simulink model "tengbeudpv1"  (Simulink 7.4)
settings: Solver=ode45  StartTime=0.0  StopTime=1000  RelTol=1e-3
libraries: xbsIndex_r4 x132, xps_library x15, casper_library_misc x6, casper_library_flow_control x4
settings Model: Creator=dsp  LastModifiedBy=gofrito  CovModelRefEnable=off
settings OptimizationCC: InitFltsAndDblsToZero=on
settings DebuggingCC: SaveWithParameterizedLinksMsg=none  SignalResolutionControl=TryResolveAllWithWarning  MultiTaskDSMMsg=warning  MultiTaskCondExecSysMsg=none  StrictBusMsg=None
settings RTWCC: IncludeERTFirstTime=on
settings GRTTargetCC: TargetFcnLib=ansi_tfl_tmw.mat

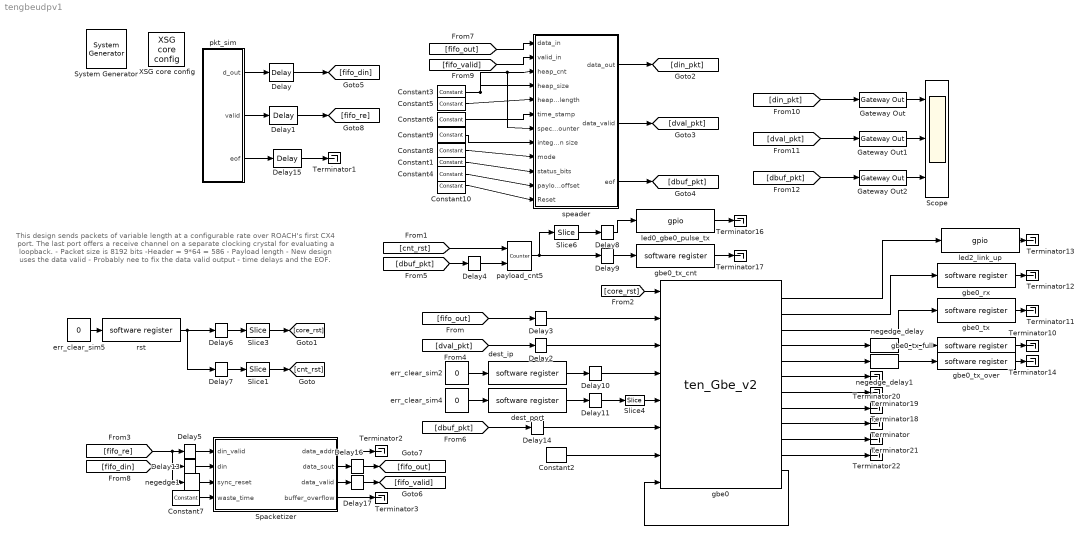
== system tengbeudpv1 ==
  note: This design sends packets of variable length at a configurable rate
      | over ROACH's first CX4 port.
      | The last port offers a receive channel on a separate
      | clocking crystal for evaluating a loopback.
      |
      | - Packet size is 8192 bits
      | -Header = 9*64 = 586
      | - Payload length
      | - New design uses the data valid
      | - Probably nee to fix the data valid output - time delays and the EOF.
  " System Generator" : xbsIndex_r4/ System Generator  Tag=genX  SystemSampleTime=-1  xilinxfamily=virtex5  part=xc5vsx95t  speed=-1  package=ff1136  synthesis_tool=XST  clock_wrapper=Clock Enables  directory=./tengbeudpv1/sysgen  testbench=off  simulink_period=1  sysclk_period=5  dcm_input_clock_period=100  incr_netlist=off  trim_vbits=Everywhere in SubSystem  dbl_ovrd=According to Block Masks  core_generation=According to Block Masks  run_coregen=off  deprecated_control=off  eval_field=0  block_type=sysgen
      settings: block_version=10.1.3
  Constant{1,4,6,8..9} (5 alike) : xbsIndex_r4/Constant  arith_type=Unsigned  const=0  n_bits=40  bin_pt=0  explicit_period=on  period=1  equ=P=C  opselect=C  inp2=PCIN>>17  opr=+  inp1=P  carry=CIN  dbl_ovrd=off  block_type=constant
  Constant10 : xbsIndex_r4/Constant  arith_type=Boolean  const=0  n_bits=40  bin_pt=0  explicit_period=on  period=1  equ=P=C  opselect=C  inp2=PCIN>>17  opr=+  inp1=P  carry=CIN  dbl_ovrd=off  block_type=constant
  Constant2 : xbsIndex_r4/Constant  arith_type=Boolean  const=1  n_bits=1  bin_pt=0  explicit_period=on  period=1  equ=P=C  opselect=C  inp2=PCIN>>17  opr=+  inp1=P  carry=CIN  dbl_ovrd=off  block_type=constant
  Constant3 : xbsIndex_r4/Constant  arith_type=Unsigned  const=128*2+6*8  n_bits=40  bin_pt=0  explicit_period=on  period=1  equ=P=C  opselect=C  inp2=PCIN>>17  opr=+  inp1=P  carry=CIN  dbl_ovrd=off  block_type=constant
  Constant5 : xbsIndex_r4/Constant  arith_type=Unsigned  const=256  n_bits=40  bin_pt=0  explicit_period=on  period=1  equ=P=C  opselect=C  inp2=PCIN>>17  opr=+  inp1=P  carry=CIN  dbl_ovrd=off  block_type=constant
  Constant7 : xbsIndex_r4/Constant  arith_type=Unsigned  const=4  n_bits=7  bin_pt=0  explicit_period=on  period=1  equ=P=C  opselect=C  inp2=PCIN>>17  opr=+  inp1=P  carry=CIN  dbl_ovrd=off  block_type=constant
  Delay{,1,4,6..11,15..17} (12 alike) : xbsIndex_r4/Delay  en=off  latency=4  dbl_ovrd=off  reg_retiming=off  block_type=delay
      settings: block_version=11.4
  Delay{2,5,13..14} (4 alike) : xbsIndex_r4/Delay  en=off  latency=2  dbl_ovrd=off  reg_retiming=off  block_type=delay
      settings: block_version=11.4
  Delay3 : xbsIndex_r4/Delay  en=off  latency=3  dbl_ovrd=off  reg_retiming=off  block_type=delay
      settings: block_version=11.4
  Gateway Out : xbsIndex_r4/Gateway Out  hdl_port=on  timing_constraint=None  locs_specified=off  LOCs={}  block_type=gatewayout
      settings: infoedit="Gateway out block.  Converts Xilinx fixed point inputs into ouputs of type Simulink integer, double, or fixed point.<br><br>Hardware notes:  In hardware these blocks become top level output ports or are discarded, depending on how they are configured."  block_version=11.4
  Gateway Out1 : xbsIndex_r4/Gateway Out  hdl_port=on  timing_constraint=None  locs_specified=off  LOCs={}  block_type=gatewayout
      settings: infoedit="Gateway out block.  Converts Xilinx fixed point inputs into ouputs of type Simulink integer, double, or fixed point.<br><br>Hardware notes:  In hardware these blocks become top level output ports or are discarded, depending on how they are configured."  block_version=11.4
  Gateway Out2 : xbsIndex_r4/Gateway Out  hdl_port=on  timing_constraint=None  locs_specified=off  LOCs={}  block_type=gatewayout
      settings: infoedit="Gateway out block.  Converts Xilinx fixed point inputs into ouputs of type Simulink integer, double, or fixed point.<br><br>Hardware notes:  In hardware these blocks become top level output ports or are discarded, depending on how they are configured."  block_version=11.4
  Scope : Scope  NumInputPorts=3
      settings: YMin=-5~-5~-5  YMax=5~5~5
  Slice1 : xbsIndex_r4/Slice  nbits=1  boolean_output=on  mode=Lower Bit Location + Width  bit1=0  base1=MSB of Input  bit0=0  base0=LSB of Input  dbl_ovrd=off  block_type=slice
      settings: infoedit="Extracts a given range of bits from each input sample and presents it at the output.  The output type is ordinarily unsigned with binary point at zero, but can be Boolean when the slice is one bit wide.<P><P>Hardware notes: In hardware this block costs nothing."  block_version=10.1.3
  Slice3 : xbsIndex_r4/Slice  nbits=1  boolean_output=on  mode=Lower Bit Location + Width  bit1=0  base1=MSB of Input  bit0=1  base0=LSB of Input  dbl_ovrd=off  block_type=slice
      settings: block_version=10.1.3
  Slice4 : xbsIndex_r4/Slice  nbits=16  boolean_output=off  mode=Lower Bit Location + Width  bit1=0  base1=MSB of Input  bit0=0  base0=LSB of Input  dbl_ovrd=off  block_type=slice
      settings: infoedit="Extracts a given range of bits from each input sample and presents it at the output.  The output type is ordinarily unsigned with binary point at zero, but can be Boolean when the slice is one bit wide.<P><P>Hardware notes: In hardware this block costs nothing."  block_version=10.1.3
  Slice6 : xbsIndex_r4/Slice  nbits=1  boolean_output=on  mode=Lower Bit Location + Width  bit1=0  base1=MSB of Input  bit0=27-12  base0=LSB of Input  dbl_ovrd=off  block_type=slice
      settings: infoedit="Extracts a given range of bits from each input sample and presents it at the output.  The output type is ordinarily unsigned with binary point at zero, but can be Boolean when the slice is one bit wide.<P><P>Hardware notes: In hardware this block costs nothing."  block_version=10.1.3
  Spacketizer : Subsystem  AncestorBlock=gbt_library/Spacketizer  mask(packetizer){pin_width=256, sout_width=64, fifo_depth=2K, total_words=32}
      mask prompts: pin_width "Parallel Input Width"; sout_width "Serial Output Width"; fifo_depth "FIFO depth"; total_words "Total number of data points"
      mask help:
      | This block is intended to serialize data that is 'bursty', that is,
      | the average data rate is small but per cycle the data is highly
      | parallel and can contain many points simultaneously.  This situation
      | is common with the streaming CASPER FFTs and related blocks.
      |
      | The serialization buffers the data when valid and independently
      | serializes the data when the buffer is non-empty.  For convenience, the
      | data is counted as it is serialized and signals exist to indicate
      | that the serial output is valid or that a buffer overflow has occured.  The
      | block will not stop in the case of an overflow, and the overflow
      | signal is not held high after it occurs.
      |
      | For example usage, see 'roach_spec_2adc_borph' in 'SVNROOT/trunk/projects/roach_spec/'
      | or the test case in 'SVNROOT/trunk/mlib_devel_10_1/Tests/packetizer_test.mdl'
      |
      | For extended documentation, please see the CASPER wiki
      mask init:
      | packetizer_init(gcb, 'pin_width', pin_width, 'sout_width', sout_width, 'total_words', total_words, 'fifo_depth', fifo_depth)
      | % packetizer_init(gcb, ...
      | %     'pin_width', pin_width, ...
      | %     'sout_width', sout_width, ...
      | %   %  'fifo_depth', fifo_depth, ...
      | %     'total_words', total_words);
      settings: AttributesFormatString=|
      | Parallel Input Width: 256
      | Serial Output Width: 64
      mask StyleString: edit,edit,popup(16|32|64|128|256|512|1K|2K|4K|8K|16K|32K|64K),edit
  Terminator{,1..3,10..14,16..22} (16 alike) : Terminator
  XSG core config : xps_library/XSG core config  Tag=xps:xsg  SystemSampleTime=-1  hw_sys=ROACH:sx95t  ibob_linux=off  clk_src=sys_clk2x  iBOB_clk_src=sys_clk  BEE2_ctrl_clk_src=sys_clk  BEE2_usr_clk_src=sys_clk  ROACH_clk_src=sys_clk2x  CORR_clk_src=sys_clk  gpio_clk_io_group=iBOB:sma  gpio_clk_bit_index=0  clk_rate=200  sample_period=1  synthesis_tool=XST  mpc_type=powerpc440_ext
  dest_ip : xps_library/software register  Tag=xps:sw_reg  SystemSampleTime=-1  io_dir=From Processor  arith_type=Unsigned  bitwidth=32  bin_pt=0  sample_period=1  gw_name=tengbeudpv1_dest_ip_user_data_out
      link override r_10gbe_demo_dest_ip_user_data_out: arith_type=Unsigned  n_bits=32  bin_pt=0  period=1
      link override r_10gbe_test_dest_ip_user_data_out: arith_type=Unsigned  n_bits=32  bin_pt=0  period=1
      link override r_xaui_test_cnt_rst_user_data_out: arith_type=Unsigned  n_bits=32  bin_pt=0  period=1
  dest_port : xps_library/software register  Tag=xps:sw_reg  SystemSampleTime=-1  io_dir=From Processor  arith_type=Unsigned  bitwidth=32  bin_pt=0  sample_period=1  gw_name=tengbeudpv1_dest_port_user_data_out
      link override r_10gbe_demo_dest_port_user_data_out: arith_type=Unsigned  n_bits=32  bin_pt=0  period=1
      link override r_10gbe_test_dest_port_user_data_out: arith_type=Unsigned  n_bits=32  bin_pt=0  period=1
      link override r_xaui_test_cnt_rst_user_data_out: arith_type=Unsigned  n_bits=32  bin_pt=0  period=1
  err_clear_sim2 : Constant  Value=0  OutDataType=sfix(16)  OutScaling=2^0
  err_clear_sim4 : Constant  Value=0  OutDataType=sfix(16)  OutScaling=2^0
  err_clear_sim5 : Constant  Value=0  OutDataType=sfix(16)  OutScaling=2^0
  gbe0 : xps_library/ten_Gbe_v2  Tag=xps:tengbe_v2  SystemSampleTime=-1  port=0  rx_dist_ram=off  large_frames=on  show_param=on  pre_emph=3  swing=800  fab_en=on  fab_mac=hex2dec('123456780000')  fab_ip=10*(2^24) + 0*(2^16) + 0*(2^8) + 20*(2^0)  fab_udp=10000  fab_gate=1  cpu_rx_en=on  cpu_tx_en=on
  gbe0_rx : xps_library/software register  Tag=xps:sw_reg  SystemSampleTime=-1  io_dir=To Processor  arith_type=Unsigned  bitwidth=32  bin_pt=0  sample_period=1  gw_name=tengbeudpv1_gbe0_rx_user_data_in
      link override convert: arith_type=Unsigned  n_bits=32  bin_pt=0
  gbe0_tx : xps_library/software register  Tag=xps:sw_reg  SystemSampleTime=-1  io_dir=To Processor  arith_type=Unsigned  bitwidth=32  bin_pt=0  sample_period=1  gw_name=tengbeudpv1_gbe0_tx_user_data_in
      link override convert: arith_type=Unsigned  n_bits=32  bin_pt=0
  gbe0_tx_cnt : xps_library/software register  Tag=xps:sw_reg  SystemSampleTime=-1  io_dir=To Processor  arith_type=Unsigned  bitwidth=32  bin_pt=0  sample_period=1  gw_name=tengbeudpv1_gbe0_tx_cnt_user_data_in
      link override convert: arith_type=Unsigned  n_bits=32  bin_pt=0
  gbe0_tx_full : xps_library/software register  Tag=xps:sw_reg  SystemSampleTime=-1  io_dir=To Processor  arith_type=Unsigned  bitwidth=32  bin_pt=0  sample_period=1  gw_name=tengbeudpv1_gbe0_tx_full_user_data_in
      link override convert: arith_type=Unsigned  n_bits=32  bin_pt=0
  gbe0_tx_over : xps_library/software register  Tag=xps:sw_reg  SystemSampleTime=-1  io_dir=To Processor  arith_type=Unsigned  bitwidth=32  bin_pt=0  sample_period=1  gw_name=tengbeudpv1_gbe0_tx_over_user_data_in
      link override convert: arith_type=Unsigned  n_bits=32  bin_pt=0
  led0_gbe0_pulse_tx : xps_library/gpio  Tag=xps:gpio  SystemSampleTime=-1  io_group=ROACH:led  io_dir=out  arith_type=Boolean  bitwidth=1  bin_pt=0  bit_index=0  sample_period=1  use_single_ended=off  use_ddr=off  reg_iob=off  reg_clk_phase=0  termination=None
      link override convert: arith_type=Boolean  n_bits=1  bin_pt=0
  led2_link_up : xps_library/gpio  Tag=xps:gpio  SystemSampleTime=-1  io_group=ROACH:led  io_dir=out  arith_type=Boolean  bitwidth=1  bin_pt=0  bit_index=2  sample_period=1  use_single_ended=off  use_ddr=off  reg_iob=off  reg_clk_phase=0  termination=None
      link override convert: arith_type=Boolean  n_bits=1  bin_pt=0
  negedge1 : casper_library_misc/negedge  Tag=Rising Edge Detector  SystemSampleTime=-1
  negedge_delay : casper_library_misc/negedge_delay  SystemSampleTime=-1  pulse_len=2^20
  negedge_delay1 : casper_library_misc/negedge_delay  SystemSampleTime=-1  pulse_len=2^20
  payload_cnt5 : xbsIndex_r4/Counter  cnt_type=Free Running  cnt_to=0  operation=Up  start_count=0  cnt_by_val=1  arith_type=Unsigned  n_bits=32  bin_pt=0  load_pin=off  rst=on  en=on  explicit_period=on  period=1  dbl_ovrd=off  use_behavioral_HDL=off  implementation=Fabric  use_rpm=on  block_type=counter
      settings: xl_area=[0, 0, 0, 0, 0, 0, 0]
  pkt_sim : Subsystem
  rst : xps_library/software register  Tag=xps:sw_reg  SystemSampleTime=-1  io_dir=From Processor  arith_type=Unsigned  bitwidth=32  bin_pt=0  sample_period=1  gw_name=tengbeudpv1_rst_user_data_out
      link override r_10gbe_demo_gbe_core_rst_user_data_out: arith_type=Unsigned  n_bits=32  bin_pt=0  period=1
      link override r_10gbe_test_cnt_rst_user_data_out: arith_type=Unsigned  n_bits=32  bin_pt=0  period=1
      link override r_10gbe_test_gbe_core_rst_user_data_out: arith_type=Unsigned  n_bits=32  bin_pt=0  period=1
      link override r_xaui_test_cnt_rst_user_data_out: arith_type=Unsigned  n_bits=32  bin_pt=0  period=1
  speader : Subsystem  AncestorBlock=gbt_library/spead_packet  mask{spead_msw=64, spead_lsw=40, num_items=6}
      mask prompts: num_items "Number of items (+5)"
      mask help:
      | The size of the heap and payload are in Bytes.
      | If there is one packet per heap then payload_offset is 0.
      | All the input must be not longer than 40 bits.
  wires:
  Constant2/1 -> gbe0/7
  err_clear_sim2/1 -> dest_ip/1
  dest_ip/1 -> Delay10/1
  err_clear_sim4/1 -> dest_port/1
  dest_port/1 -> Delay11/1
  Slice4/1 -> gbe0/5
  gbe0/12 -> gbe0/8
  gbe0/5 -> negedge_delay1/1
  gbe0/1 -> led2_link_up/1
  gbe0/2 -> gbe0_rx/1
  gbe0/3 -> gbe0_tx/1
  gbe0/4 -> negedge_delay/1
  negedge_delay1/1 -> gbe0_tx_over/1
  negedge_delay/1 -> gbe0_tx_full/1
  payload_cnt5/1 -> Slice6/1, Delay9/1
  Slice6/1 -> Delay8/1
  err_clear_sim5/1 -> rst/1
  rst/1 -> Delay6/1, Delay7/1
  Slice1/1 -> [cnt_rst]
  [cnt_rst] -> payload_cnt5/1
  Slice3/1 -> [core_rst]
  [core_rst] -> gbe0/1
  gbe0/9 -> Terminator/1
  led2_link_up/1 -> Terminator13/1
  gbe0_rx/1 -> Terminator12/1
  gbe0_tx/1 -> Terminator11/1
  gbe0_tx_full/1 -> Terminator10/1
  gbe0_tx_over/1 -> Terminator14/1
  led0_gbe0_pulse_tx/1 -> Terminator16/1
  gbe0_tx_cnt/1 -> Terminator17/1
  gbe0/11 -> Terminator22/1
  gbe0/10 -> Terminator21/1
  gbe0/8 -> Terminator18/1
  gbe0/7 -> Terminator19/1
  gbe0/6 -> Terminator20/1
  pkt_sim/2(valid) -> Delay1/1
  Delay6/1 -> Slice3/1
  Delay7/1 -> Slice1/1
  Delay8/1 -> led0_gbe0_pulse_tx/1
  Delay9/1 -> gbe0_tx_cnt/1
  Delay10/1 -> gbe0/4
  Delay11/1 -> Slice4/1
  [fifo_out] -> Delay3/1
  [dval_pkt] -> Delay2/1
  Delay4/1 -> payload_cnt5/2
  [dbuf_pkt] -> Delay4/1
  Delay14/1 -> gbe0/6
  Delay2/1 -> gbe0/3
  Delay3/1 -> gbe0/2
  pkt_sim/3(eof) -> Delay15/1
  [dbuf_pkt] -> Delay14/1
  pkt_sim/1(d_out) -> Delay/1
  Delay15/1 -> Terminator1/1
  Constant3/1 -> speader/4(heap_size), speader/3(heap_cnt), speader/7(spectrum counter)
  Constant5/1 -> speader/5(heap_pay_length)
  speader/1(data_out) -> [din_pkt]
  speader/2(data_valid) -> [dval_pkt]
  speader/3(eof) -> [dbuf_pkt]
  Constant6/1 -> speader/6(time_stamp)
  [fifo_out] -> speader/1(data_in)
  Delay1/1 -> [fifo_re]
  [fifo_valid] -> speader/2(valid_in)
  Constant1/1 -> speader/10(status_bits)
  Constant4/1 -> speader/11(payload_offset)
  Constant9/1 -> speader/8(integration size)
  Constant8/1 -> speader/9(mode)
  Constant10/1 -> speader/12(Reset)
  Gateway Out/1 -> Scope/1
  [din_pkt] -> Gateway Out/1
  Gateway Out1/1 -> Scope/2
  [dval_pkt] -> Gateway Out1/1
  Gateway Out2/1 -> Scope/3
  [dbuf_pkt] -> Gateway Out2/1
  Delay/1 -> [fifo_din]
  Spacketizer/1(data_addr) -> Terminator2/1
  Spacketizer/2(data_sout) -> Delay16/1
  Spacketizer/3(data_valid) -> Delay17/1
  Spacketizer/4(buffer_overflow) -> Terminator3/1
  Constant7/1 -> Spacketizer/4(waste_time)
  [fifo_re] -> Delay5/1, negedge1/1
  [fifo_din] -> Delay13/1
  negedge1/1 -> Spacketizer/3(sync_reset)
  Delay5/1 -> Spacketizer/1(din_valid)
  Delay13/1 -> Spacketizer/2(din)
  Delay16/1 -> [fifo_out]
  Delay17/1 -> [fifo_valid]

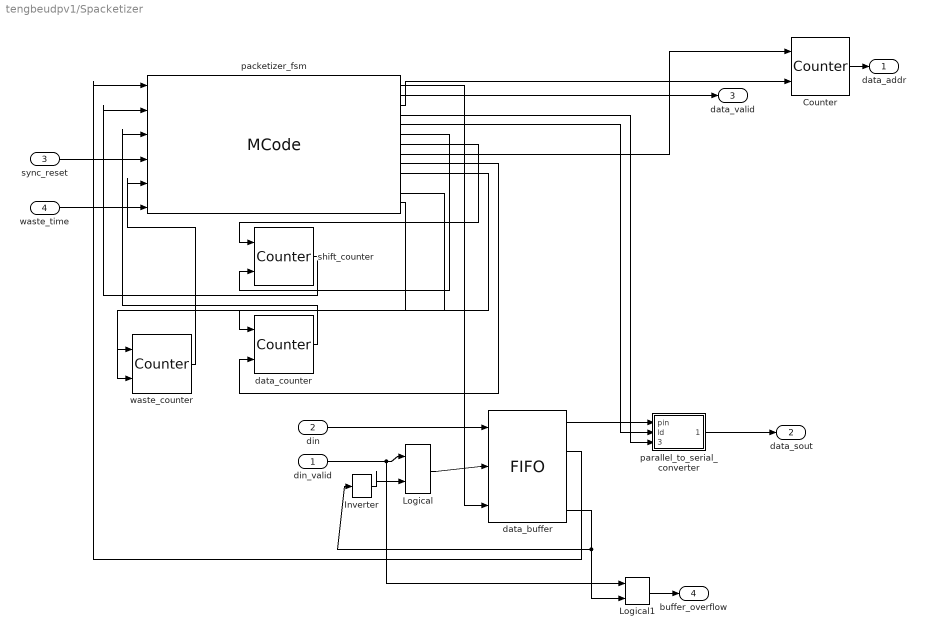
== system tengbeudpv1/Spacketizer ==
  din_valid : Inport
  din : Inport  Port=2
  sync_reset : Inport  Port=3
  waste_time : Inport  Port=4
  Counter : xbsIndex_r4/Counter  cnt_type=Free Running  cnt_to=Inf  operation=Up  start_count=0  cnt_by_val=1  arith_type=Unsigned  n_bits=11  bin_pt=0  load_pin=off  rst=on  en=on  explicit_period=on  period=1  dbl_ovrd=off  use_behavioral_HDL=off  implementation=Fabric  use_rpm=off  block_type=counter
  Inverter : xbsIndex_r4/Inverter  en=off  latency=0  dbl_ovrd=off  block_type=inv
  Logical : xbsIndex_r4/Logical  logical_function=AND  inputs=2  en=off  latency=0  precision=Full  arith_type=Unsigned  n_bits=16  bin_pt=0  align_bp=on  dbl_ovrd=off  block_type=logical
  Logical1 : xbsIndex_r4/Logical  logical_function=AND  inputs=2  en=off  latency=0  precision=Full  arith_type=Unsigned  n_bits=16  bin_pt=0  align_bp=on  dbl_ovrd=off  block_type=logical
  data_buffer : xbsIndex_r4/FIFO  depth=2K  percent_nbits=1  rst=off  en=off  use_dcount=off  use_almost_empty=off  almost_empty_thresh=2  use_almost_full=off  almost_full_thresh=14  dbl_ovrd=off  mem_type=Block RAM  explicit_period=off  block_type=fifo
      settings: block_version=10.1.3
  data_counter : xbsIndex_r4/Counter  cnt_type=Free Running  cnt_to=Inf  operation=Up  start_count=0  cnt_by_val=1  arith_type=Unsigned  n_bits=6  bin_pt=0  load_pin=off  rst=on  en=on  explicit_period=on  period=1  dbl_ovrd=off  use_behavioral_HDL=off  implementation=Fabric  use_rpm=off  block_type=counter
  packetizer_fsm : xbsIndex_r4/MCode  mfname=packetizer_fsm  explicit_period=off  period=1  inputsTable={'boundInpExpr'=>['','','3','',' 31 ','','',''],'inputs'=>['fifo_empty','shift_count','data_per_word','data_count','n_words','sync_reset','waste_count','waste_time']}  outputsTable={'outputs'=>['fifo_re','bram_addr_en','bram_we','serializer_shift','serializer_ld','shift_count_en','shift_count_rst','bram_addr_rst','data_count_en','data_count_rst','done','waste_count_en','waste_count_rst'],'suppressOut'=>['off','off','off','off','off','off','off','off','off','off','off','off','off']}  dbl_ovrd=off  enable_stdout=off  enable_debug=off  suppress_output=on  defparams={'data_per_word',3, 'n_words', 31 }  hide_port_list={}  block_type=mcode
      settings: block_version=11.4
  parallel_to_serial_converter : Subsystem  AncestorBlock=casper_library/Flow_Control/parallel_to_serial_converter  mask(parallel_to_serial_converter){pin_width=256, sout_width=64}
      mask prompts: pin_width "Parallel Input Width"; sout_width "Serial Output Width"
      mask help:
      | This block takes as input a parallel bus of specified width.
      | When the load signal 'ld' is asserted, this data is broken into
      | pieces of width specified by the serial output width and
      | stored into different registers chained to form a shift register.
      | If the 'shift' input is subsequently asserted, the shift register
      | returns as output a new piece of data of width sout_width.  This data
      | is the next least significant piece of the original bus.  The converter
      | serializes SMALL ENDIAN.
      |
      | Note that the load operation automatically loads the least significant
      | bits into the register closest to the output, so the first 'shift'
      | assertion changes the data output from bits [sout_width-1:0] to
      | bits [2*sout_width-1:sout_width].
      mask init:
      | parallel_to_serial_converter_init(gcb, ...
      |     'pin_width', pin_width, ...
      |     'sout_width', sout_width);
  shift_counter : xbsIndex_r4/Counter  cnt_type=Free Running  cnt_to=Inf  operation=Up  start_count=0  cnt_by_val=1  arith_type=Unsigned  n_bits=3  bin_pt=0  load_pin=off  rst=on  en=on  explicit_period=on  period=1  dbl_ovrd=off  use_behavioral_HDL=off  implementation=Fabric  use_rpm=off  block_type=counter
  waste_counter : xbsIndex_r4/Counter  cnt_type=Free Running  cnt_to=Inf  operation=Up  start_count=0  cnt_by_val=1  arith_type=Unsigned  n_bits=5  bin_pt=0  load_pin=off  rst=on  en=on  explicit_period=on  period=1  dbl_ovrd=off  use_behavioral_HDL=off  implementation=Fabric  use_rpm=off  block_type=counter
  data_addr : Outport
  data_sout : Outport  Port=2
  data_valid : Outport  Port=3
  buffer_overflow : Outport  Port=4
  wires:
  Logical1/1 -> buffer_overflow/1
  data_buffer/4 -> Logical1/2, Inverter/1
  Inverter/1 -> Logical/2
  din_valid/1 -> Logical1/1, Logical/1
  Logical/1 -> data_buffer/2
  data_buffer/1 -> parallel_to_serial_converter/1(pin)
  packetizer_fsm/1 -> data_buffer/3
  packetizer_fsm/4 -> parallel_to_serial_converter/3(shift)
  packetizer_fsm/5 -> parallel_to_serial_converter/2(ld)
  packetizer_fsm/3 -> data_valid/1
  din/1 -> data_buffer/1
  parallel_to_serial_converter/1(sout) -> data_sout/1
  packetizer_fsm/6 -> shift_counter/2
  shift_counter/1 -> packetizer_fsm/2
  packetizer_fsm/7 -> shift_counter/1
  data_buffer/2 -> packetizer_fsm/1
  Counter/1 -> data_addr/1
  packetizer_fsm/2 -> Counter/2
  packetizer_fsm/8 -> Counter/1
  packetizer_fsm/9 -> data_counter/2
  data_counter/1 -> packetizer_fsm/3
  packetizer_fsm/10 -> data_counter/1
  sync_reset/1 -> packetizer_fsm/4
  waste_counter/1 -> packetizer_fsm/5
  packetizer_fsm/12 -> waste_counter/2
  packetizer_fsm/13 -> waste_counter/1
  waste_time/1 -> packetizer_fsm/6

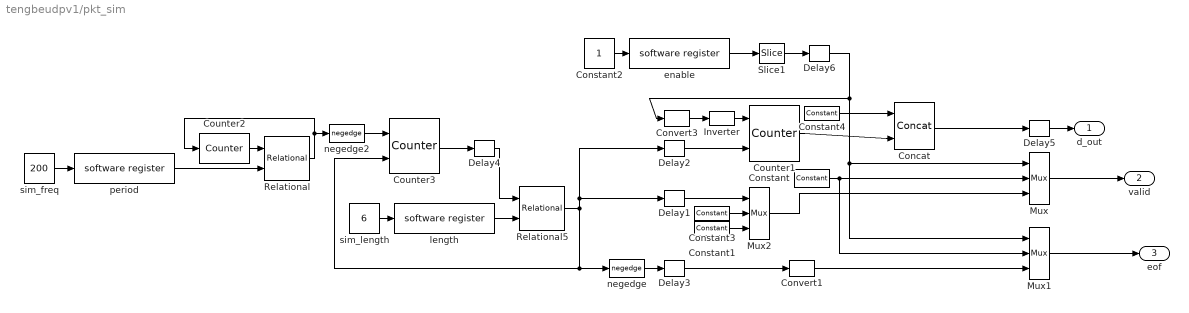
== system tengbeudpv1/pkt_sim ==
  Concat : xbsIndex_r4/Concat  num_inputs=2  dbl_ovrd=off  block_type=concat
  Constant : xbsIndex_r4/Constant  arith_type=Boolean  const=0  n_bits=1  bin_pt=0  explicit_period=on  period=1  equ=P=C  opselect=C  inp2=PCIN>>17  opr=+  inp1=P  carry=CIN  dbl_ovrd=off  block_type=constant
  Constant1 : xbsIndex_r4/Constant  arith_type=Boolean  const=1  n_bits=1  bin_pt=0  explicit_period=off  period=1  equ=P=C  opselect=C  inp2=PCIN>>17  opr=+  inp1=P  carry=CIN  dbl_ovrd=off  block_type=constant
  Constant2 : Constant  OutDataType=sfix(16)  OutScaling=2^0
  Constant3 : xbsIndex_r4/Constant  arith_type=Boolean  const=0  n_bits=1  bin_pt=0  explicit_period=off  period=1  equ=P=C  opselect=C  inp2=PCIN>>17  opr=+  inp1=P  carry=CIN  dbl_ovrd=off  block_type=constant
  Constant4 : xbsIndex_r4/Constant  arith_type=Unsigned  const=0  n_bits=256-32  bin_pt=0  explicit_period=off  period=1  equ=P=C  opselect=C  inp2=PCIN>>17  opr=+  inp1=P  carry=CIN  dbl_ovrd=off  block_type=constant
  Convert1 : xbsIndex_r4/Convert  arith_type=Boolean  n_bits=8  bin_pt=6  quantization=Truncate  overflow=Wrap  latency=0  dbl_ovrd=off  pipeline=off  block_type=convert
      settings: xl_area=[0, 0, 0, 0, 0, 0, 0]  block_version=10.1.3
  Convert3 : xbsIndex_r4/Convert  arith_type=Boolean  n_bits=8  bin_pt=6  quantization=Truncate  overflow=Wrap  latency=0  dbl_ovrd=off  pipeline=off  block_type=convert
      settings: xl_area=[0, 0, 0, 0, 0, 0, 0]  block_version=10.1.3
  Counter1 : xbsIndex_r4/Counter  cnt_type=Free Running  cnt_to=Inf  operation=Up  start_count=0  cnt_by_val=1  arith_type=Unsigned  n_bits=32  bin_pt=0  load_pin=off  rst=on  en=on  explicit_period=off  period=1  dbl_ovrd=off  use_behavioral_HDL=off  implementation=Fabric  use_rpm=off  block_type=counter
      settings: xl_area=[0, 0, 0, 0, 0, 0, 0]
  Counter2 : xbsIndex_r4/Counter  cnt_type=Free Running  cnt_to=Inf  operation=Up  start_count=1  cnt_by_val=1  arith_type=Unsigned  n_bits=32  bin_pt=0  load_pin=off  rst=on  en=off  explicit_period=on  period=1  dbl_ovrd=off  use_behavioral_HDL=off  implementation=Fabric  use_rpm=on  block_type=counter
      settings: xl_area=[0, 0, 0, 0, 0, 0, 0]
  Counter3 : xbsIndex_r4/Counter  cnt_type=Free Running  cnt_to=1023  operation=Up  start_count=0  cnt_by_val=1  arith_type=Unsigned  n_bits=32  bin_pt=0  load_pin=off  rst=on  en=on  explicit_period=on  period=1  dbl_ovrd=off  use_behavioral_HDL=off  implementation=Fabric  use_rpm=on  block_type=counter
      settings: xl_area=[0, 0, 0, 0, 0, 0, 0]
  Delay1 : xbsIndex_r4/Delay  en=off  latency=3  dbl_ovrd=off  reg_retiming=on  block_type=delay
      settings: xl_area=[0, 0, 0, 0, 0, 0, 0]
  Delay2 : xbsIndex_r4/Delay  en=off  latency=3  dbl_ovrd=off  reg_retiming=on  block_type=delay
      settings: xl_area=[0, 0, 0, 0, 0, 0, 0]
  Delay3 : xbsIndex_r4/Delay  en=off  latency=3  dbl_ovrd=off  reg_retiming=on  block_type=delay
      settings: xl_area=[0, 0, 0, 0, 0, 0, 0]
  Delay4 : xbsIndex_r4/Delay  en=off  latency=2  dbl_ovrd=off  reg_retiming=on  block_type=delay
      settings: xl_area=[0, 0, 0, 0, 0, 0, 0]
  Delay5 : xbsIndex_r4/Delay  en=off  latency=2  dbl_ovrd=off  reg_retiming=on  block_type=delay
      settings: xl_area=[0, 0, 0, 0, 0, 0, 0]
  Delay6 : xbsIndex_r4/Delay  en=off  latency=2  dbl_ovrd=off  reg_retiming=on  block_type=delay
      settings: xl_area=[0, 0, 0, 0, 0, 0, 0]
  Inverter : xbsIndex_r4/Inverter  en=off  latency=0  dbl_ovrd=off  block_type=inv
      settings: xl_area=[0, 0, 0, 0, 0, 0, 0]
  Mux : xbsIndex_r4/Mux  inputs=2  en=off  latency=2  precision=Full  arith_type="Signed  (2's comp)"  n_bits=8  bin_pt=2  quantization=Truncate  overflow=Wrap  dbl_ovrd=off  block_type=mux
      settings: xl_area=[0, 0, 0, 0, 0, 0, 0]
  Mux1 : xbsIndex_r4/Mux  inputs=2  en=off  latency=2  precision=Full  arith_type="Signed  (2's comp)"  n_bits=8  bin_pt=2  quantization=Truncate  overflow=Wrap  dbl_ovrd=off  block_type=mux
      settings: xl_area=[0, 0, 0, 0, 0, 0, 0]
  Mux2 : xbsIndex_r4/Mux  inputs=2  en=off  latency=1  precision=Full  arith_type="Signed  (2's comp)"  n_bits=8  bin_pt=2  quantization=Truncate  overflow=Wrap  dbl_ovrd=off  block_type=mux
      settings: xl_area=[0, 0, 0, 0, 0, 0, 0]
  Relational : xbsIndex_r4/Relational  mode=a>=b  en=off  latency=0  dbl_ovrd=off  block_type=relational
      settings: xl_area=[0, 0, 0, 0, 0, 0, 0]  block_version=10.1.3
  Relational5 : xbsIndex_r4/Relational  mode=a<b  en=off  latency=0  dbl_ovrd=off  block_type=relational
      settings: xl_area=[0, 0, 0, 0, 0, 0, 0]  block_version=10.1.3
  Slice1 : xbsIndex_r4/Slice  nbits=1  boolean_output=off  mode=Lower Bit Location + Width  bit1=1  base1=MSB of Input  bit0=0  base0=LSB of Input  dbl_ovrd=off  block_type=slice
      settings: block_version=10.1.3
  enable : xps_library/software register  Tag=xps:sw_reg  SystemSampleTime=-1  io_dir=From Processor  arith_type=Unsigned  bitwidth=32  bin_pt=0  sample_period=1  gw_name=tengbeudpv1_pkt_sim_enable_user_data_out
      link override r_10gbe_demo_pkt_sim_run_user_data_out: arith_type=Unsigned  n_bits=32  bin_pt=0  period=1
      link override r_10gbe_test_pkt_sim_run_user_data_out: arith_type=Unsigned  n_bits=32  bin_pt=0  period=1
      link override test_pkt_buffer_10_1_p_mux_up_run_user_data_out: arith_type=Unsigned  n_bits=32  bin_pt=0  period=1
  length : xps_library/software register  Tag=xps:sw_reg  SystemSampleTime=-1  io_dir=From Processor  arith_type=Unsigned  bitwidth=32  bin_pt=0  sample_period=1  gw_name=tengbeudpv1_pkt_sim_length_user_data_out
      link override r_10gbe_demo_pkt_sim_payload_len_user_data_out: arith_type=Unsigned  n_bits=32  bin_pt=0  period=1
      link override r_10gbe_test_pkt_sim_payload_len_user_data_out: arith_type=Unsigned  n_bits=32  bin_pt=0  period=1
      link override test_pkt_buffer_10_1_p_mux_up_payload_len_user_data_out: arith_type=Unsigned  n_bits=32  bin_pt=0  period=1
  negedge : casper_library_misc/negedge  Tag=Rising Edge Detector  SystemSampleTime=-1
  negedge2 : casper_library_misc/negedge  Tag=Rising Edge Detector  SystemSampleTime=-1
  period : xps_library/software register  Tag=xps:sw_reg  SystemSampleTime=-1  io_dir=From Processor  arith_type=Unsigned  bitwidth=32  bin_pt=0  sample_period=1  gw_name=tengbeudpv1_pkt_sim_period_user_data_out
      link override r_10gbe_demo_pkt_sim_period_user_data_out: arith_type=Unsigned  n_bits=32  bin_pt=0  period=1
      link override r_10gbe_test_pkt_sim_period_user_data_out: arith_type=Unsigned  n_bits=32  bin_pt=0  period=1
      link override test_pkt_buffer_10_1_p_mux_up_period_user_data_out: arith_type=Unsigned  n_bits=32  bin_pt=0  period=1
  sim_freq : Constant  Value=200  OutDataType=sfix(16)  OutScaling=2^0
  sim_length : Constant  Value=6  OutDataType=sfix(16)  OutScaling=2^0
  d_out : Outport  OutDataType=sfix(16)  OutScaling=2^0
  valid : Outport  Port=2  OutDataType=sfix(16)  OutScaling=2^0
  eof : Outport  Port=3  OutDataType=sfix(16)  OutScaling=2^0
  wires:
  Counter2/1 -> Relational/1
  Relational/1 -> Counter2/1, negedge2/1
  negedge/1 -> Delay3/1
  period/1 -> Relational/2
  sim_freq/1 -> period/1
  Relational5/1 -> Counter3/2, negedge/1, Delay1/1, Delay2/1
  Counter3/1 -> Delay4/1
  negedge2/1 -> Counter3/1
  sim_length/1 -> length/1
  length/1 -> Relational5/2
  Mux/1 -> valid/1
  Constant/1 -> Mux/2, Mux1/2
  Mux1/1 -> eof/1
  Delay3/1 -> Convert1/1
  Convert1/1 -> Mux1/3
  Delay5/1 -> d_out/1
  enable/1 -> Slice1/1
  Constant2/1 -> enable/1
  Slice1/1 -> Delay6/1
  Mux2/1 -> Mux/3
  Inverter/1 -> Counter1/1
  Delay2/1 -> Counter1/2
  Convert3/1 -> Inverter/1
  Constant3/1 -> Mux2/2
  Constant1/1 -> Mux2/3
  Delay1/1 -> Mux2/1
  Delay4/1 -> Relational5/1
  Delay6/1 -> Mux/1, Mux1/1, Convert3/1
  Concat/1 -> Delay5/1
  Counter1/1 -> Concat/2
  Constant4/1 -> Concat/1

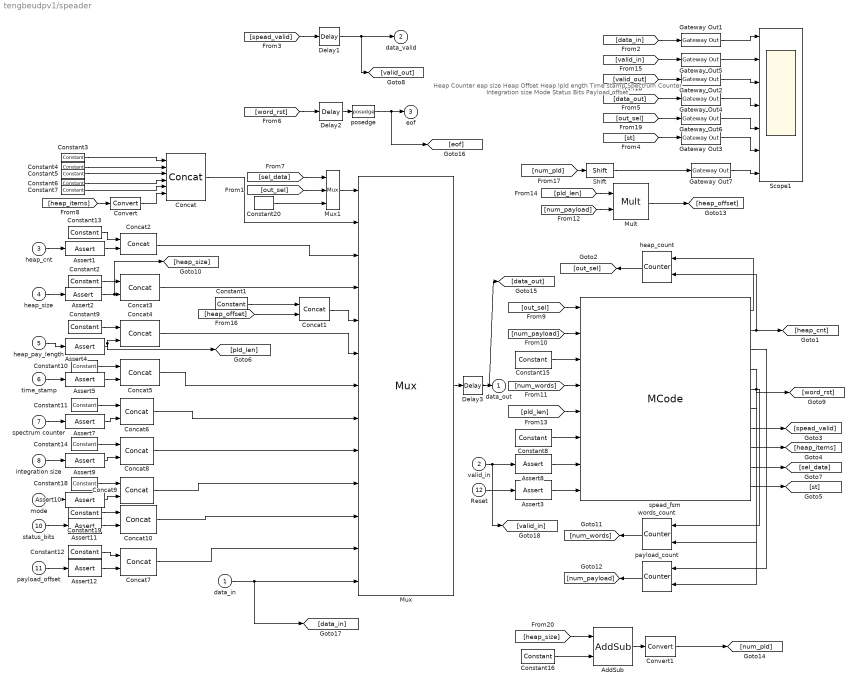
== system tengbeudpv1/speader ==
  note: Heap Counter
      | eap size
      | Heap Offset
      | Heap lpld ength
      | Time stamp
      | Spectrum Counter
      | Integration size
      | Mode
      | Status Bits
      | Payload offset
  data_in : Inport
  valid_in : Inport  Port=2
  heap_cnt : Inport  Port=3
  heap_size : Inport  Port=4
  heap_pay_length : Inport  Port=5
  time_stamp : Inport  Port=6
  spectrum counter : Inport  Port=7
  integration size : Inport  Port=8
  mode : Inport  Port=9
  status_bits : Inport  Port=10
  payload_offset : Inport  Port=11
  Reset : Inport  Port=12
  AddSub : xbsIndex_r4/AddSub  mode=Subtraction  use_carryin=off  use_carryout=off  en=off  latency=0  precision=User Defined  arith_type=Unsigned  n_bits=40  bin_pt=0  quantization=Truncate  overflow=Wrap  dbl_ovrd=off  use_behavioral_HDL=off  hw_selection=Fabric  pipelined=off  block_type=addsub
  Assert{1..2,4..5,7,9..12} (9 alike) : xbsIndex_r4/Assert  assert_type=on  type_source=Explicitly  arith_type=Unsigned  n_bits=spead_lsw  bin_pt=0  assert_rate=off  rate_source=Explicitly  period=1  output_port=on  block_type=assert
      settings: block_version=11.4
  Assert3 : xbsIndex_r4/Assert  assert_type=on  type_source=Explicitly  arith_type=Boolean  n_bits=spead_lsw  bin_pt=0  assert_rate=on  rate_source=Explicitly  period=1  output_port=on  block_type=assert
      settings: block_version=11.4
  Assert8 : xbsIndex_r4/Assert  assert_type=on  type_source=Explicitly  arith_type=Boolean  n_bits=spead_lsw  bin_pt=0  assert_rate=on  rate_source=Explicitly  period=1  output_port=on  block_type=assert
      settings: block_version=11.4
  Concat : xbsIndex_r4/Concat  num_inputs=6  dbl_ovrd=off  block_type=concat
  Concat{1..10} (10 alike) : xbsIndex_r4/Concat  num_inputs=2  dbl_ovrd=off  block_type=concat
  Constant1 : xbsIndex_r4/Constant  arith_type=Unsigned  const=8388611  n_bits=spead_msw-spead_lsw  bin_pt=0  explicit_period=on  period=1  equ=P=C  opselect=C  inp2=PCIN>>17  opr=+  inp1=P  carry=CIN  dbl_ovrd=off  block_type=constant
      settings: block_version=11.4
  Constant10 : xbsIndex_r4/Constant  arith_type=Unsigned  const=8388628  n_bits=spead_msw-spead_lsw  bin_pt=0  explicit_period=on  period=1  equ=P=C  opselect=C  inp2=PCIN>>17  opr=+  inp1=P  carry=CIN  dbl_ovrd=off  block_type=constant
      settings: block_version=11.4
  Constant11 : xbsIndex_r4/Constant  arith_type=Unsigned  const=8388629  n_bits=spead_msw-spead_lsw  bin_pt=0  explicit_period=on  period=1  equ=P=C  opselect=C  inp2=PCIN>>17  opr=+  inp1=P  carry=CIN  dbl_ovrd=off  block_type=constant
      settings: block_version=11.4
  Constant12 : xbsIndex_r4/Constant  arith_type=Unsigned  const=26  n_bits=spead_msw-spead_lsw  bin_pt=0  explicit_period=on  period=1  equ=P=C  opselect=C  inp2=PCIN>>17  opr=+  inp1=P  carry=CIN  dbl_ovrd=off  block_type=constant
      settings: block_version=11.4
  Constant13 : xbsIndex_r4/Constant  arith_type=Unsigned  const=8388609  n_bits=spead_msw-spead_lsw  bin_pt=0  explicit_period=on  period=1  equ=P=C  opselect=C  inp2=PCIN>>17  opr=+  inp1=P  carry=CIN  dbl_ovrd=off  block_type=constant
      settings: block_version=11.4
  Constant14 : xbsIndex_r4/Constant  arith_type=Unsigned  const=8388630  n_bits=spead_msw-spead_lsw  bin_pt=0  explicit_period=on  period=1  equ=P=C  opselect=C  inp2=PCIN>>17  opr=+  inp1=P  carry=CIN  dbl_ovrd=off  block_type=constant
      settings: block_version=11.4
  Constant15 : xbsIndex_r4/Constant  arith_type=Unsigned  const=num_items+5  n_bits=8  bin_pt=0  explicit_period=on  period=1  equ=P=C  opselect=C  inp2=PCIN>>17  opr=+  inp1=P  carry=CIN  dbl_ovrd=off  block_type=constant
      settings: block_version=11.4
  Constant16 : xbsIndex_r4/Constant  arith_type=Unsigned  const=num_items*8  n_bits=8  bin_pt=0  explicit_period=on  period=1  equ=P=C  opselect=C  inp2=PCIN>>17  opr=+  inp1=P  carry=CIN  dbl_ovrd=off  block_type=constant
      settings: block_version=11.4
  Constant18 : xbsIndex_r4/Constant  arith_type=Unsigned  const=8388631  n_bits=spead_msw-spead_lsw  bin_pt=0  explicit_period=on  period=1  equ=P=C  opselect=C  inp2=PCIN>>17  opr=+  inp1=P  carry=CIN  dbl_ovrd=off  block_type=constant
      settings: block_version=11.4
  Constant19 : xbsIndex_r4/Constant  arith_type=Unsigned  const=8388632  n_bits=spead_msw-spead_lsw  bin_pt=0  explicit_period=on  period=1  equ=P=C  opselect=C  inp2=PCIN>>17  opr=+  inp1=P  carry=CIN  dbl_ovrd=off  block_type=constant
      settings: block_version=11.4
  Constant2 : xbsIndex_r4/Constant  arith_type=Unsigned  const=8388610  n_bits=spead_msw-spead_lsw  bin_pt=0  explicit_period=on  period=1  equ=P=C  opselect=C  inp2=PCIN>>17  opr=+  inp1=P  carry=CIN  dbl_ovrd=off  block_type=constant
      settings: block_version=11.4
  Constant20 : xbsIndex_r4/Constant  arith_type=Unsigned  const=num_items+5  n_bits=4  bin_pt=0  explicit_period=on  period=1  equ=P=C  opselect=C  inp2=PCIN>>17  opr=+  inp1=P  carry=CIN  dbl_ovrd=off  block_type=constant
      settings: block_version=11.4
  Constant3 : xbsIndex_r4/Constant  arith_type=Unsigned  const=83  n_bits=8  bin_pt=0  explicit_period=on  period=1  equ=P=C  opselect=C  inp2=PCIN>>17  opr=+  inp1=P  carry=CIN  dbl_ovrd=off  block_type=constant
      settings: block_version=11.4
  Constant4 : xbsIndex_r4/Constant  arith_type=Unsigned  const=4  n_bits=8  bin_pt=0  explicit_period=on  period=1  equ=P=C  opselect=C  inp2=PCIN>>17  opr=+  inp1=P  carry=CIN  dbl_ovrd=off  block_type=constant
      settings: block_version=11.4
  Constant5 : xbsIndex_r4/Constant  arith_type=Unsigned  const=3  n_bits=8  bin_pt=0  explicit_period=on  period=1  equ=P=C  opselect=C  inp2=PCIN>>17  opr=+  inp1=P  carry=CIN  dbl_ovrd=off  block_type=constant
      settings: block_version=11.4
  Constant6 : xbsIndex_r4/Constant  arith_type=Unsigned  const=5  n_bits=8  bin_pt=0  explicit_period=on  period=1  equ=P=C  opselect=C  inp2=PCIN>>17  opr=+  inp1=P  carry=CIN  dbl_ovrd=off  block_type=constant
      settings: block_version=11.4
  Constant7 : xbsIndex_r4/Constant  arith_type=Unsigned  const=0  n_bits=16  bin_pt=0  explicit_period=on  period=1  equ=P=C  opselect=C  inp2=PCIN>>17  opr=+  inp1=P  carry=CIN  dbl_ovrd=off  block_type=constant
      settings: block_version=11.4
  Constant8 : xbsIndex_r4/Constant  arith_type=Unsigned  const=2  n_bits=8  bin_pt=0  explicit_period=on  period=1  equ=P=C  opselect=C  inp2=PCIN>>17  opr=+  inp1=P  carry=CIN  dbl_ovrd=off  block_type=constant
      settings: block_version=11.4
  Constant9 : xbsIndex_r4/Constant  arith_type=Unsigned  const=8388612  n_bits=spead_msw-spead_lsw  bin_pt=0  explicit_period=on  period=1  equ=P=C  opselect=C  inp2=PCIN>>17  opr=+  inp1=P  carry=CIN  dbl_ovrd=off  block_type=constant
      settings: block_version=11.4
  Convert : xbsIndex_r4/Convert  arith_type=Unsigned  n_bits=16  bin_pt=0  quantization=Truncate  overflow=Wrap  latency=0  dbl_ovrd=off  pipeline=off  block_type=convert
      settings: block_version=11.4
  Convert1 : xbsIndex_r4/Convert  arith_type=Unsigned  n_bits=16  bin_pt=0  quantization=Truncate  overflow=Wrap  latency=0  dbl_ovrd=off  pipeline=off  block_type=convert
      settings: block_version=11.4
  Delay1 : xbsIndex_r4/Delay  en=off  latency=1  dbl_ovrd=off  reg_retiming=on  block_type=delay
      settings: block_version=11.4
  Delay2 : xbsIndex_r4/Delay  en=off  latency=0  dbl_ovrd=off  reg_retiming=on  block_type=delay
      settings: block_version=11.4
  Delay3 : xbsIndex_r4/Delay  en=off  latency=1  dbl_ovrd=off  reg_retiming=on  block_type=delay
      settings: block_version=11.4
  Gateway Out{1..7} (7 alike) : xbsIndex_r4/Gateway Out  hdl_port=on  timing_constraint=None  locs_specified=off  LOCs={}  block_type=gatewayout
      settings: infoedit="Gateway out block.  Converts Xilinx fixed point inputs into ouputs of type Simulink integer, double, or fixed point.<br><br>Hardware notes:  In hardware these blocks become top level output ports or are discarded, depending on how they are configured."  block_version=11.4
  Mult : xbsIndex_r4/Mult  precision=User Defined  arith_type=Unsigned  n_bits=40  bin_pt=0  quantization=Truncate  overflow=Wrap  en=off  latency=3  dbl_ovrd=off  use_behavioral_HDL=off  opt=Speed  use_embedded=on  optimum_pipeline=off  pipeline=on  use_rpm=on  placement_style=Triangular  block_type=mult
      settings: block_version=11.4
  Mux : xbsIndex_r4/Mux  inputs=12  en=off  latency=0  precision=User Defined  arith_type=Unsigned  n_bits=64  bin_pt=0  quantization=Truncate  overflow=Wrap  dbl_ovrd=off  block_type=mux
      settings: block_version=11.4
  Mux1 : xbsIndex_r4/Mux  inputs=2  en=off  latency=0  precision=Full  arith_type="Signed  (2's comp)"  n_bits=8  bin_pt=2  quantization=Truncate  overflow=Wrap  dbl_ovrd=off  block_type=mux
      settings: block_version=11.4
  Scope1 : Scope  NumInputPorts=7
      settings: TimeRange=1000  YMin=0~0~0~0~0~0~-5  YMax=40~1~1~1e+19~1~20~5  SaveName=ScopeData2  MaxDataPoints=10000
  Shift : xbsIndex_r4/Shift  shift_dir=Right  shift_bits=2  en=off  latency=0  precision=Full  arith_type="Signed  (2's comp)"  n_bits=16  bin_pt=14  quantization=Truncate  overflow=Wrap  dbl_ovrd=off  block_type=shift
  heap_count : xbsIndex_r4/Counter  cnt_type=Free Running  cnt_to=Inf  operation=Up  start_count=0  cnt_by_val=1  arith_type=Unsigned  n_bits=4  bin_pt=0  load_pin=off  rst=on  en=on  explicit_period=on  period=1  dbl_ovrd=off  use_behavioral_HDL=off  implementation=Fabric  block_type=counter
      settings: block_version=11.4
  payload_count : xbsIndex_r4/Counter  cnt_type=Free Running  cnt_to=Inf  operation=Up  start_count=0  cnt_by_val=1  arith_type=Unsigned  n_bits=8  bin_pt=0  load_pin=off  rst=on  en=on  explicit_period=on  period=1  dbl_ovrd=off  use_behavioral_HDL=off  implementation=Fabric  block_type=counter
      settings: block_version=11.4
  posedge : casper_library_misc/posedge  Tag=Rising Edge Detector  SystemSampleTime=-1
  spead_fsm : xbsIndex_r4/MCode  mfname=spead_fsm  explicit_period=on  period=1  inputsTable={'boundInpExpr'=>['','','','5','','','','',''],'inputs'=>['head_count','num_payload_sent','total_header_len','min_header_len','num_words_sent','payload_len','total_num_payloads','data_valid_in','rst']}  outputsTable={'outputs'=>['head_count_rst','head_count_en','num_payload_rst','num_payload_en','words_sent_rst','words_sent_en','tge_valid','heap_elements','select_data','st'],'suppressOut'=>['off','off','off','off','off','off','off','off','off','off']}  dbl_ovrd=off  enable_stdout=off  enable_debug=off  suppress_output=on  defparams={'min_header_len',5}  hide_port_list={}  block_type=mcode
      settings: block_version=11.4
  words_count : xbsIndex_r4/Counter  cnt_type=Free Running  cnt_to=Inf  operation=Up  start_count=0  cnt_by_val=8  arith_type=Unsigned  n_bits=10  bin_pt=0  load_pin=off  rst=on  en=on  explicit_period=on  period=1  dbl_ovrd=off  use_behavioral_HDL=off  implementation=Fabric  block_type=counter
      settings: block_version=11.4
  data_out : Outport
  data_valid : Outport  Port=2
  eof : Outport  Port=3
  wires:
  Assert12/1 -> Concat7/2
  payload_offset/1 -> Assert12/1
  Assert11/1 -> Concat10/2
  status_bits/1 -> Assert11/1
  Constant19/1 -> Concat10/1
  Assert10/1 -> Concat9/2
  mode/1 -> Assert10/1
  Constant18/1 -> Concat9/1
  Concat4/1 -> Mux/6
  Concat3/1 -> Mux/4
  Concat/1 -> Mux/2
  Constant9/1 -> Concat4/1
  Constant7/1 -> Concat/5
  Constant6/1 -> Concat/4
  Constant5/1 -> Concat/3
  Constant4/1 -> Concat/2
  Constant3/1 -> Concat/1
  Constant2/1 -> Concat3/1
  Constant13/1 -> Concat2/1
  Constant12/1 -> Concat7/1
  Constant10/1 -> Concat5/1
  data_in/1 -> [data_in], Mux/13
  time_stamp/1 -> Assert5/1
  heap_size/1 -> Assert2/1
  heap_cnt/1 -> Assert1/1
  Assert1/1 -> Concat2/2
  Assert2/1 -> Concat3/2, [heap_size]
  Assert4/1 -> Concat4/2, [pld_len]
  Assert5/1 -> Concat5/2
  Concat2/1 -> Mux/3
  [spead_valid] -> Delay1/1
  heap_pay_length/1 -> Assert4/1
  [valid_out] -> Gateway Out2/1
  Delay1/1 -> data_valid/1, [valid_out]
  [out_sel] -> Gateway Out6/1
  Constant1/1 -> Concat1/1
  Concat1/1 -> Mux/5
  Concat7/1 -> Mux/12
  Concat10/1 -> Mux/11
  Concat9/1 -> Mux/10
  spectrum counter/1 -> Assert7/1
  Assert7/1 -> Concat6/2
  Constant11/1 -> Concat6/1
  Concat6/1 -> Mux/8
  Concat5/1 -> Mux/7
  integration size/1 -> Assert9/1
  Assert9/1 -> Concat8/2
  Constant14/1 -> Concat8/1
  Concat8/1 -> Mux/9
  Gateway Out2/1 -> Scope1/3
  Gateway Out6/1 -> Scope1/5
  spead_fsm/5 -> words_count/1
  spead_fsm/6 -> words_count/2
  spead_fsm/3 -> payload_count/1
  spead_fsm/4 -> payload_count/2, [word_rst]
  spead_fsm/1 -> heap_count/1
  spead_fsm/2 -> heap_count/2, [heap_cnt]
  spead_fsm/7 -> [spead_valid]
  spead_fsm/8 -> [heap_items]
  valid_in/1 -> Assert8/1, [valid_in]
  [heap_offset] -> Concat1/2
  Reset/1 -> Assert3/1
  [data_in] -> Gateway Out1/1
  Gateway Out1/1 -> Scope1/1
  Gateway Out3/1 -> Scope1/6
  Gateway Out4/1 -> Scope1/4
  [data_out] -> Gateway Out4/1
  Constant20/1 -> Mux1/3
  Mux1/1 -> Mux/1
  spead_fsm/10 -> [st]
  spead_fsm/9 -> [sel_data]
  [heap_items] -> Convert/1
  Convert/1 -> Concat/6
  words_count/1 -> [num_words]
  payload_count/1 -> [num_payload]
  heap_count/1 -> [out_sel]
  [out_sel] -> spead_fsm/1
  [num_payload] -> spead_fsm/2
  [valid_in] -> Gateway Out5/1
  Gateway Out5/1 -> Scope1/2
  posedge/1 -> eof/1, [eof]
  [word_rst] -> Delay2/1
  Assert3/1 -> spead_fsm/8
  Assert8/1 -> spead_fsm/7
  Constant8/1 -> spead_fsm/6
  [pld_len] -> spead_fsm/5
  [num_words] -> spead_fsm/4
  Constant15/1 -> spead_fsm/3
  Delay2/1 -> posedge/1
  [heap_size] -> AddSub/1
  Constant16/1 -> AddSub/2
  AddSub/1 -> Convert1/1
  Convert1/1 -> [num_pld]
  [num_payload] -> Mult/2
  [pld_len] -> Mult/1
  Mult/1 -> [heap_offset]
  Delay3/1 -> data_out/1, [data_out]
  Mux/1 -> Delay3/1
  [out_sel] -> Mux1/2
  [sel_data] -> Mux1/1
  [st] -> Gateway Out3/1
  [num_pld] -> Shift/1
  Gateway Out7/1 -> Scope1/7
  Shift/1 -> Gateway Out7/1

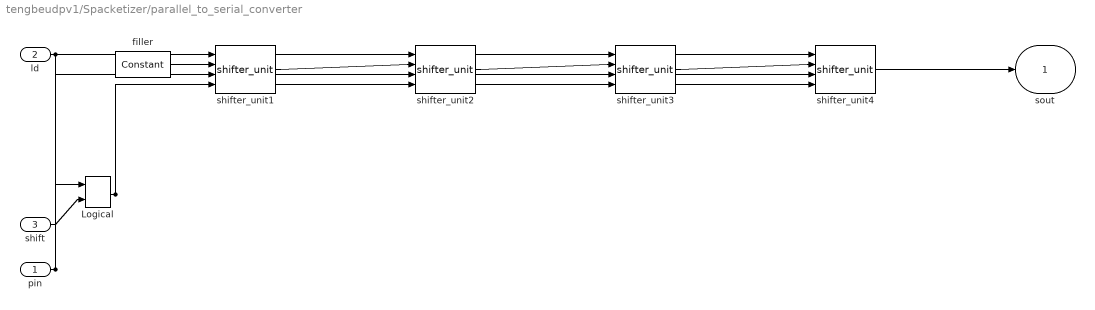
== system tengbeudpv1/Spacketizer/parallel_to_serial_converter ==
  pin : Inport
  ld : Inport  Port=2
  shift : Inport  Port=3
  Logical : xbsIndex_r4/Logical  logical_function=OR  inputs=2  en=off  latency=0  precision=Full  arith_type=Unsigned  n_bits=16  bin_pt=0  align_bp=on  dbl_ovrd=off  block_type=logical
  filler : xbsIndex_r4/Constant  arith_type=Unsigned  const=0  n_bits=sout_width  bin_pt=0  explicit_period=on  period=1  equ=P=C  opselect=C  inp2=PCIN>>17  opr=+  inp1=P  carry=CIN  dbl_ovrd=off  block_type=constant
  shifter_unit1 : casper_library_flow_control/shifter_unit  SystemSampleTime=-1  data_width=64  pin_offset=0
  shifter_unit2 : casper_library_flow_control/shifter_unit  SystemSampleTime=-1  data_width=64  pin_offset=64
  shifter_unit3 : casper_library_flow_control/shifter_unit  SystemSampleTime=-1  data_width=64  pin_offset=128
  shifter_unit4 : casper_library_flow_control/shifter_unit  SystemSampleTime=-1  data_width=64  pin_offset=192
  sout : Outport  OutDataType=sfix(16)  OutScaling=2^0
  wires:
  ld/1 -> Logical/1, shifter_unit1/1, shifter_unit2/1, shifter_unit3/1, shifter_unit4/1
  shift/1 -> Logical/2
  filler/1 -> shifter_unit1/2
  pin/1 -> shifter_unit1/3, shifter_unit2/3, shifter_unit3/3, shifter_unit4/3
  Logical/1 -> shifter_unit1/4, shifter_unit2/4, shifter_unit3/4, shifter_unit4/4
  shifter_unit1/1 -> shifter_unit2/2
  shifter_unit2/1 -> shifter_unit3/2
  shifter_unit3/1 -> shifter_unit4/2
  shifter_unit4/1 -> sout/1
